simulink model "SynGen_transient_stability"  (R2018a)
settings: Solver=VariableStepAuto  StartTime=0.0  StopTime=2  RelTol=1e-3
libraries: powerlib x10, powerlib_meascontrol x4
settings Model: Creator=acs-mmi  LastModifiedBy=acs-mmi

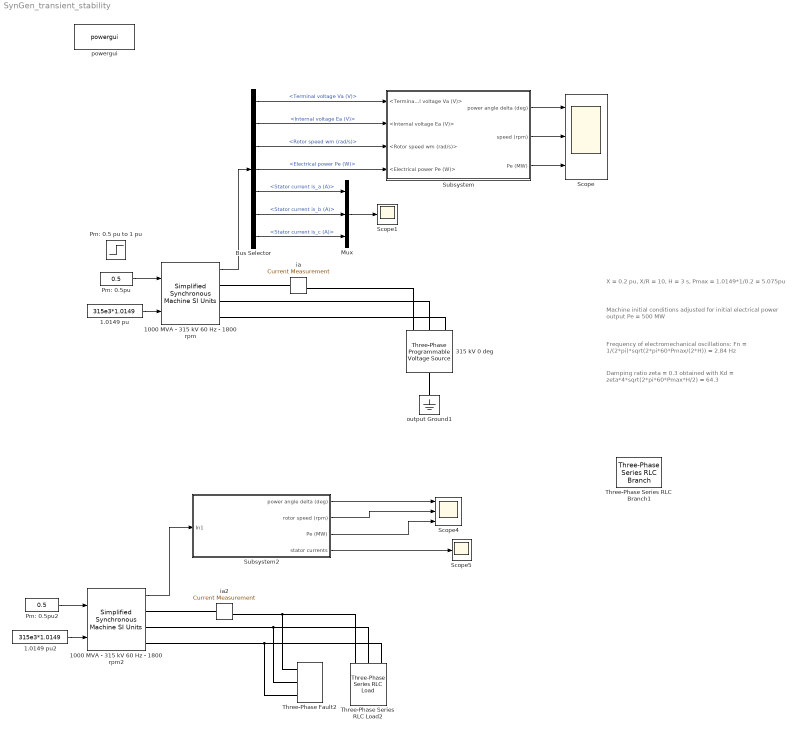
== system SynGen_transient_stability ==
  note: Machine  initial conditions adjusted
      | for initial  electrical power output Pe = 500 MW
  note: X = 0.2 pu, X/R = 10, H = 3 s, Pmax = 1.0149*1/0.2 = 5.075pu
  note: Frequency of electromechanical oscillations:
      | Fn = 1/(2*pi)*sqrt(2*pi*60*Pmax/(2*H)) = 2.84 Hz
  note: Damping ratio zeta = 0.3 obtained with
      | Kd = zeta*4*sqrt(2*pi*60*Pmax*H/2) = 64.3
  1.0149 pu : Constant  Value=315e3*1.0149
  1.0149 pu2 : Constant  Value=315e3*1.0149
  1000 MVA - 315 kV 60 Hz - 1800 rpm : powerlib/Machines/Simplified Synchronous Machine SI Units  ConnectionType=3-wire Y  MechanicalLoad=Mechanical power Pm  MeasurementBus=off  NominalParameters=[ 1000e6, 315e3, 60 ]  Mechanical="[168870,  64.3,  2]"  InternalRL=[ 99.225*0.02 ,99.225/(2*pi*60)*0.2 ]  InitialConditions=[0 5.65442 1296.03 1296.03 1296.03 0 -120 120]  Units=1  LoadFlowParameters=[1 500000000 0 0 0]  TsPowergui=0  TsBlock=-1  BusType=PV  Pref=0  Qref=0  Qmin=-inf  Qmax=+inf  PLF=0  QLF=0
      settings: AttributesFormatString=\n  SourceProductName=Simscape Power Systems  SourceProductBaseCode=PS
  1000 MVA - 315 kV 60 Hz - 1800 rpm2 : powerlib/Machines/Simplified Synchronous Machine SI Units  ConnectionType=3-wire Y  MechanicalLoad=Mechanical power Pm  MeasurementBus=off  NominalParameters=[ 1000e6, 315e3, 60 ]  Mechanical="[168870,  64.3,  2]"  InternalRL=[ 99.225*0.02 ,99.225/(2*pi*60)*0.2 ]  InitialConditions=[0 5.65442 1296.03 1296.03 1296.03 0 -120 120]  Units=1  LoadFlowParameters=[1 500000000 0 0 0]  TsPowergui=0  TsBlock=-1  BusType=PV  Pref=0  Qref=0  Qmin=-inf  Qmax=+inf  PLF=0  QLF=0
      settings: AttributesFormatString=\n  SourceProductName=Simscape Power Systems  SourceProductBaseCode=PS
  315 kV 0 deg : powerlib/Electrical Sources/Three-Phase Programmable Voltage Source  PositiveSequence="[315e3 0  60]"  VariationEntity=None  VariationType=Step  VariationTypeAlt=Step  VariationStep=-0.5  VariationRate=10  VariationMagnitude=0.3  VariationFrequency=2  VariationTiming=[0.1 1.2]  VariationPhaseA=off  Amplitudes=[1 0.8 1.2 1.0]  TimeValues=[0 0.1 0.15 0.2]  HarmonicGeneration=off  HarmonicA=[3 0.2 -25 0]  HarmonicB="[2 0.15  35 2]"  Timing="[0.05  3]"  BusType=swing  Pref=0  Qref=0  Qmin=-inf  Qmax=inf
  Bus Selector : BusSelector  OutputSignals=Terminal voltage Va (V),Internal voltage Ea (V),Rotor speed wm (rad/s),Electrical power Pe (W),Stator current is_a (A),Stator current is_b (A),Stator current is_c (A)
  Mux : Mux  Inputs=3
  Pm: 0.5 pu to 1 pu : Step  Time=0.5  Before=505e6  After=1000e6  SampleTime=0
  Pm: 0.5pu : Constant  Value=0.5
  Pm: 0.5pu2 : Constant  Value=0.5
  Scope : Scope  NumInputPorts=3
  Scope1 : Scope
  Scope4 : Scope  NumInputPorts=3
  Scope5 : Scope
  Subsystem : Subsystem
  Subsystem2 : Subsystem
  Three-Phase Series RLC Branch1 : powerlib/Elements/Three-Phase Series RLC Branch  LConnTagsString=A|B|C  RConnTagsString=A|B|C  BranchType=RLC  Resistance=1  Inductance=1e-3  Capacitance=1e-6  Measurements=None
  Three-Phase Series RLC Load2 : powerlib/Elements/Three-Phase Series RLC Load  LConnTagsString=A|B|C  Configuration=Y (grounded)  NominalVoltage=315e3  Vabc=[1e3 1e3 1e3]  Vabcp=[1e3 1e3 1e3]  NominalFrequency=60  UnbalancedPower=off  ActivePower=100e6  InductivePower=0  CapacitivePower=0  Pabc=[10e3 9e3 11e3]  QLabc=[100 90 110]  QCabc=[100 90 110]  Pabcp=[10e3 9e3 11e3]  QLabcp=[100 90 110]  QCabcp=[100 90 110]  Measurements=None  LoadType=constant Z
  Three-Phase Fault2 : powerlib/Elements/Three-Phase Fault  InitialStates=0  FaultA=on  FaultB=on  FaultC=on  GroundFault=on  SwitchTimes="[1  1.5]"  External=off  SwitchStatus=NaN  FaultResistance=0.0001  GroundResistance=10  SnubberResistance=1e6  SnubberCapacitance=inf  Measurements=None
  ia : powerlib/Measurements/Current Measurement  Tag=PoWeRsYsTeMmEaSuReMeNt  PhasorSimulation=off  OutputType=Magnitude  PSBequivalent=0
  ia2 : powerlib/Measurements/Current Measurement  Tag=PoWeRsYsTeMmEaSuReMeNt  PhasorSimulation=off  OutputType=Magnitude  PSBequivalent=0
  output Ground1 : powerlib/Elements/Ground  LConnTagsString=a
  powergui : powerlib/powergui  Priority=2  SimulationMode=Continuous  SampleTime=0  frequency=60  Iterations=50  frequencyindice=60  Pbase=100e6  ErrMax=1e-4  UnitsV=kV  UnitsW=MW  buscounter=0  FunctionMessages=off  echomessages=off  EnableUseOfTLC=off  CurrentSourceSwitches=off  DisableSnubberDevices=off  DisableRonSwitches=off  DisableVfSwitches=off  DisplayEquations=off  SolverType=Tustin/Backward Euler (TBE)  Interpol=off  ExternalGateDelay=off  methode=off  Ts=100  x0status=blocks  SPID=off  SwTol=0  HookPort=off  RestoreLinks=warning  ResistiveCurrentMeasurement=off  Frange=[0:2:500]  Ylog=off  Xlog=off  ShowGrid=off  save=off  variable=ZData  structure=0  ZoomFFT=on  StartTime=0.0  cycles=1  DisplayStyle=off  fundamental=60  FreqAxis=off  MaxFrequency=1000  frequencyindicesteady=1  RmsSteady=1  display=off
  wires:
  1000 MVA - 315 kV 60 Hz - 1800 rpm/1 -> Bus Selector/1
  1.0149 pu/1 -> 1000 MVA - 315 kV 60 Hz - 1800 rpm/2
  Pm: 0.5pu/1 -> 1000 MVA - 315 kV 60 Hz - 1800 rpm/1
  Bus Selector/1 -> Subsystem/1(<Terminal voltage Va (V)>)  "<Terminal voltage Va (V)>"
  Bus Selector/2 -> Subsystem/2(<Internal voltage Ea (V)>)  "<Internal voltage Ea (V)>"
  Bus Selector/3 -> Subsystem/3(<Rotor speed wm (rad/s)>)  "<Rotor speed wm (rad/s)>"
  Bus Selector/4 -> Subsystem/4(<Electrical power Pe (W)>)  "<Electrical power Pe (W)>"
  Subsystem/1(power angle delta (deg)) -> Scope/1
  Subsystem/2(speed (rpm)) -> Scope/2
  Subsystem/3(Pe (MW)) -> Scope/3
  Mux/1 -> Scope1/1
  Bus Selector/5 -> Mux/1  "<Stator current is_a (A)>"
  Bus Selector/6 -> Mux/2  "<Stator current is_b (A)>"
  Bus Selector/7 -> Mux/3  "<Stator current is_c (A)>"
  1.0149 pu2/1 -> 1000 MVA - 315 kV 60 Hz - 1800 rpm2/2
  Pm: 0.5pu2/1 -> 1000 MVA - 315 kV 60 Hz - 1800 rpm2/1
  1000 MVA - 315 kV 60 Hz - 1800 rpm2/1 -> Subsystem2/1(In1)
  Subsystem2/1(power angle delta (deg)) -> Scope4/1
  Subsystem2/2(rotor speed (rpm)) -> Scope4/2
  Subsystem2/3(Pe (MW)) -> Scope4/3
  Subsystem2/4(stator currents) -> Scope5/1
  connections:
  315 kV 0 deg/LConn1 -- output Ground1/LConn1
  315 kV 0 deg/RConn1 -- ia/RConn1
  1000 MVA - 315 kV 60 Hz - 1800 rpm/RConn1 -- ia/LConn1
  315 kV 0 deg/RConn3 -- 1000 MVA - 315 kV 60 Hz - 1800 rpm/RConn3
  315 kV 0 deg/RConn2 -- 1000 MVA - 315 kV 60 Hz - 1800 rpm/RConn2
  Three-Phase Series RLC Load2/LConn1 -- ia2/RConn1 -- Three-Phase Fault2/LConn1
  Three-Phase Series RLC Load2/LConn2 -- 1000 MVA - 315 kV 60 Hz - 1800 rpm2/RConn2 -- Three-Phase Fault2/LConn2
  Three-Phase Series RLC Load2/LConn3 -- 1000 MVA - 315 kV 60 Hz - 1800 rpm2/RConn3 -- Three-Phase Fault2/LConn3
  1000 MVA - 315 kV 60 Hz - 1800 rpm2/RConn1 -- ia2/LConn1

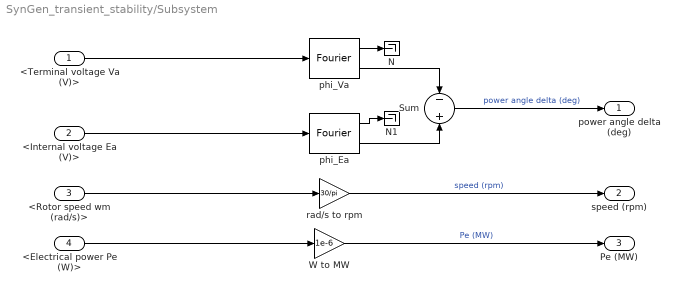
== system SynGen_transient_stability/Subsystem ==
  <Terminal voltage Va (V)> : Inport
  <Internal voltage Ea (V)> : Inport  Port=2
  <Rotor speed wm (rad/s)> : Inport  Port=3
  <Electrical power Pe (W)> : Inport  Port=4
  N : Terminator
  N1 : Terminator
  Sum : Sum  Inputs=-+  SaturateOnIntegerOverflow=on  InputSameDT=on  OutDataTypeStr=Inherit: Same as first input
  W to MW : Gain  Gain=1e-6  SaturateOnIntegerOverflow=on  OutDataTypeStr=Inherit: Same as input  ParamDataTypeStr=Inherit: Same as input
  phi_Ea : powerlib_meascontrol/Measurements/Fourier  Freq=60  n=1  InInit=[0, 0]  Ts=0
      settings: SourceProductName=Simscape Power Systems
  phi_Va : powerlib_meascontrol/Measurements/Fourier  Freq=60  n=1  InInit=[0, 0]  Ts=0
      settings: SourceProductName=Simscape Power Systems
  rad/s to rpm : Gain  Gain=30/pi  SaturateOnIntegerOverflow=on  OutDataTypeStr=Inherit: Same as input  ParamDataTypeStr=Inherit: Same as input
  power angle delta (deg) : Outport
  speed (rpm) : Outport  Port=2
  Pe (MW) : Outport  Port=3
  wires:
  <Terminal voltage Va (V)>/1 -> phi_Va/1
  phi_Ea/1 -> N1/1
  Sum/1 -> power angle delta (deg)/1  "power angle delta (deg)"
  phi_Va/1 -> N/1
  phi_Ea/2 -> Sum/2
  phi_Va/2 -> Sum/1
  <Rotor speed wm (rad/s)>/1 -> rad/s to rpm/1
  <Electrical power Pe (W)>/1 -> W to MW/1
  W to MW/1 -> Pe (MW)/1  "Pe (MW)"
  rad/s to rpm/1 -> speed (rpm)/1  "speed (rpm)"
  <Internal voltage Ea (V)>/1 -> phi_Ea/1

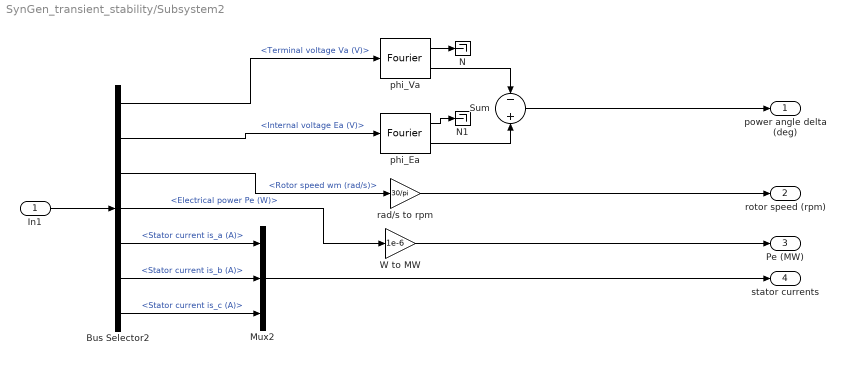
== system SynGen_transient_stability/Subsystem2 ==
  In1 : Inport
  Bus Selector2 : BusSelector  OutputSignals=Terminal voltage Va (V),Internal voltage Ea (V),Rotor speed wm (rad/s),Electrical power Pe (W),Stator current is_a (A),Stator current is_b (A),Stator current is_c (A)
  Mux2 : Mux  Inputs=3
  N : Terminator
  N1 : Terminator
  Sum : Sum  Inputs=-+  SaturateOnIntegerOverflow=on  InputSameDT=on  OutDataTypeStr=Inherit: Same as first input
  W to MW : Gain  Gain=1e-6  SaturateOnIntegerOverflow=on  OutDataTypeStr=Inherit: Same as input  ParamDataTypeStr=Inherit: Same as input
  phi_Ea : powerlib_meascontrol/Measurements/Fourier  Freq=60  n=1  InInit=[0, 0]  Ts=0
      settings: SourceProductName=Simscape Power Systems
  phi_Va : powerlib_meascontrol/Measurements/Fourier  Freq=60  n=1  InInit=[0, 0]  Ts=0
      settings: SourceProductName=Simscape Power Systems
  rad/s to rpm : Gain  Gain=30/pi  SaturateOnIntegerOverflow=on  OutDataTypeStr=Inherit: Same as input  ParamDataTypeStr=Inherit: Same as input
  power angle delta (deg) : Outport
  rotor speed (rpm) : Outport  Port=2
  Pe (MW) : Outport  Port=3
  stator currents : Outport  Port=4
  wires:
  phi_Ea/2 -> Sum/2
  Bus Selector2/6 -> Mux2/2  "<Stator current is_b (A)>"
  W to MW/1 -> Pe (MW)/1
  Bus Selector2/3 -> rad/s to rpm/1  "<Rotor speed wm (rad/s)>"
  Bus Selector2/1 -> phi_Va/1  "<Terminal voltage Va (V)>"
  phi_Ea/1 -> N1/1
  phi_Va/2 -> Sum/1
  Bus Selector2/2 -> phi_Ea/1  "<Internal voltage Ea (V)>"
  Bus Selector2/4 -> W to MW/1  "<Electrical power Pe (W)>"
  phi_Va/1 -> N/1
  Bus Selector2/7 -> Mux2/3  "<Stator current is_c (A)>"
  Bus Selector2/5 -> Mux2/1  "<Stator current is_a (A)>"
  Sum/1 -> power angle delta (deg)/1
  rad/s to rpm/1 -> rotor speed (rpm)/1
  Mux2/1 -> stator currents/1
  In1/1 -> Bus Selector2/1
